simulink model "threelevel_evenorderel_SVPWM_working"  (R2016a)
settings: Solver=VariableStepAuto  StartTime=0.0  StopTime=0.1  RelTol=1e-3
libraries: powerlib x33, simulink x7
(part 2 of 2)

== matlab function threelevel_evenorderel_SVPWM_working/Ta, Tb, Tc calc1 ==
  data: Sa1 output; Sa2 output; Sb1 output; Sb2 output; Vd input; ma input; fundf input; swf input; time input; Sc1 output; Sc2 output
function [Sa1, Sa2, Sb1, Sb2, Sc1, Sc2] = fcn(Vd,ma,fundf, swf, time)
% this program works for magnitude of Vref is greater then Vd/3 meaning ma
% must be greater than 1/sqrt(3). for smaller ma's computation is a bit
% more tricky therefore it is omitted for simplicity for now. 
%#ok<*NASGU>
Vref = ma*Vd/sqrt(3); %magnitude of Vref
theta = 2*pi*fundf*time; %angle of Vref
angle = mod(theta, 2*pi);
Ts = 1/swf;
Ta = 0;
Tb = 0;
Tc = 0;
output = 0;
Sector1 = 0; Sector2 = 0; Sector3 = 0; Sector4= 0; Sector5 = 0; Sector6 = 0;
rgn2a = 0 ;rgn2b = 0; rgn3 = 0; rgn4 = 0;
Sa1=0; Sa2=0; Sa1P=0; Sa2P=0; Sb1=0; Sb2=0; Sb1P=0; Sb2P=0; Sc1=0; Sc2=0; Sc1P=0; Sc2P=0;
anglefrom3to2= 0 ;
timee = mod(time, Ts);

%% Sector 1


if (mod(theta, 2*pi)<=pi/3)&&(mod(theta, 2*pi)>0)  % sector 1

    n = 1;
    thetaprime = angle - (n-1)*pi/3;
        for aci = 0:0.00001:pi/3   
            la = sqrt(3)*cos(aci)-sin(aci);
                if (la*ma > 0.99)&&(la*ma<=1)
                    anglefrom3to2 = aci; %leaving angle from region 3 to region 2
                    break
                end
        end

    %anglefrom3to2 = asin(1-1/(sqrt(3)*ma)); 
    anglefrom2to4 = pi/3 - anglefrom3to2; %leaving angle from region 2 to region 4
    if (mod(theta, 2*pi)<=anglefrom3to2) % then sector 1 region 3
        rgn2a = 0 ;rgn2b = 0; rgn3 = 1; rgn4 = 0;
        Ta = Ts*(2-2*ma*sin(pi/3+thetaprime));
        Tb = Ts*2*ma*sin(thetaprime);
        Tc = Ts*(2*ma*sin(pi/3-thetaprime)-1);  
        times = [Tc/4 Tb/2 Ta/2 Tc/2 Ta/2 Tb/2 Tc/4];
        times = cumsum(times);
        va1 = [1 1 1 0 1 1 1];
        va2 = [1 1 1 1 1 1 1];
        vb1 = [0 0 0 0 0 0 0];
        vb2 = [1 1 0 0 0 1 1];
        vc1 = [0 0 0 0 0 0 0];
        vc2 = [1 0 0 0 0 0 1];
        for j = 1:7
            
            if(timee<times(j))
                break
            end
        end
        Sa1=va1(j); Sa2=va2(j);
        Sb1=vb1(j); Sb2=vb2(j); 
        Sc1=vc1(j); Sc2=vc2(j); 
    else if (mod(theta,2*pi)>anglefrom3to2)&&(mod(theta,2*pi)<=anglefrom2to4) % then sector 1 region 2
            if angle<= pi/6 % then 2a
                rgn2a= 1; rgn2b = 0; rgn3 = 0; rgn4=0;
            else % then 2b
                rgn2a= 0; rgn2b = 1; rgn3 = 0; rgn4=0;
            end
            Ta = Ts*(1-2*ma*sin(thetaprime));
            Tb = Ts*(2*ma*sin(pi/3+thetaprime)-1);
            Tc = Ts*(1-2*ma*sin(pi/3-thetaprime));  
            times = [Tc/4 Tb/2 Ta/2 Tc/2 Ta/2 Tb/2 Tc/4];
            times = cumsum(times);
        if(rgn2a)
            va1 = [1 1 0 0 0 1 1];
            va2 = [1 1 1 1 1 1 1];
            vb1 = [0 0 0 0 0 0 0];
            vb2 = [1 1 1 0 1 1 1];
            vc1 = [0 0 0 0 0 0 0];
            vc2 = [1 0 0 0 0 0 1];
        for j = 1:7
            if(timee<times(j))
                break
            end
        end
        Sa1=va1(j); Sa2=va2(j);
        Sb1=vb1(j); Sb2=vb2(j); 
        Sc1=vc1(j); Sc2=vc2(j); 
        end
        if(rgn2b)
            va1 = [0 1 1 1 1 1 0];
            va2 = [1 1 1 1 1 1 1];
            vb1 = [0 0 0 1 0 0 0];
            vb2 = [1 1 1 1 1 1 1];
            vc1 = [0 0 0 0 0 0 0];
            vc2 = [0 0 1 1 1 0 0];
        for j = 1:7
            if(timee<times(j))
                break
            end
        end
        Sa1=va1(j); Sa2=va2(j);
        Sb1=vb1(j); Sb2=vb2(j); 
        Sc1=vc1(j); Sc2=vc2(j);     
        end
            
        else if (mod(theta,2*pi)>anglefrom2to4) % then sector 1 region 4
               rgn2a = 0 ;rgn2b = 0; rgn3 = 0; rgn4 = 1;
               Ta = Ts*(2*ma*sin(thetaprime)-1);
               Tb = Ts*(2*ma*sin(pi/3-thetaprime));
               Tc = Ts*(2-2*ma*sin(pi/3+thetaprime));  
               times = [Tc/4 Tb/2 Ta/2 Tc/2 Ta/2 Tb/2 Tc/4];
               times = cumsum(times);
        va1 = [0 1 1 1 1 1 0];
        va2 = [1 1 1 1 1 1 1];
        vb1 = [0 0 1 1 1 0 0];
        vb2 = [1 1 1 1 1 1 1];
        vc1 = [0 0 0 0 0 0 0];
        vc2 = [0 0 0 1 0 0 0];
        for j = 1:7
            if(timee<times(j))
                break
            end
        end
        Sa1=va1(j); Sa2=va2(j);
        Sb1=vb1(j); Sb2=vb2(j); 
        Sc1=vc1(j); Sc2=vc2(j);
            end
        end
    end
    Sector1 = 1; Sector2 = 0; Sector3 = 0; Sector4= 0; Sector5 = 0; Sector6 = 0;
end
%% Sector 2


if (mod(theta, 2*pi)<=2*pi/3)&&(mod(theta, 2*pi)>pi/3)  % sector 2
    
    n = 2;
    thetaprime = angle - (n-1)*pi/3;
        for aci = 0:0.00001:pi/3   
            la = sqrt(3)*cos(aci)-sin(aci);
                if (la*ma > 0.99)&&(la*ma<=1)
                    anglefrom3to2 = aci+pi/3; %leaving angle from region 3 to region 2
                    break
                end
        end
    %anglefrom3to2 = pi/3 + asin(1-1/(sqrt(3)*ma));
    anglefrom2to4 = pi/3 + pi/3 - anglefrom3to2;
    if (mod(theta, 2*pi)<=anglefrom3to2) % then sector 2 region 3
        rgn2a = 0 ;rgn2b = 0; rgn3 = 1; rgn4 = 0;
        Ta = Ts*(2-2*ma*sin(pi/3+thetaprime));
        Tb = Ts*2*ma*sin(thetaprime);
        Tc = Ts*(2*ma*sin(pi/3-thetaprime)-1);
        times = [Tc/4 Tb/2 Ta/2 Tc/2 Ta/2 Tb/2 Tc/4];
        times = cumsum(times);
        va1 = [0 0 1 1 1 0 0];
        va2 = [1 1 1 1 1 1 1];
        vb1 = [0 1 1 1 1 1 0];
        vb2 = [1 1 1 1 1 1 1];
        vc1 = [0 0 0 0 0 0 0];
        vc2 = [0 0 0 1 0 0 0];
        for j = 1:7
            if(timee<times(j))
                break
            end
        end
        Sa1=va1(j); Sa2=va2(j);
        Sb1=vb1(j); Sb2=vb2(j); 
        Sc1=vc1(j); Sc2=vc2(j);
    else if (mod(theta,2*pi)>anglefrom3to2)&&(mod(theta,2*pi)<=anglefrom2to4) % then sector 2 region 2
            if angle<=pi/2 %then 2a
                rgn2a= 1; rgn2b = 0; rgn3 = 0; rgn4=0;
            else % then 2b
                rgn2a= 0; rgn2b = 1; rgn3 = 0; rgn4=0;
            end
            Ta = Ts*(1-2*ma*sin(thetaprime));
            Tb = Ts*(2*ma*sin(pi/3+thetaprime)-1);
            Tc = Ts*(1-2*ma*sin(pi/3-thetaprime)); 
            times = [Tc/4 Tb/2 Ta/2 Tc/2 Ta/2 Tb/2 Tc/4];
            times = cumsum(times);
        if(rgn2a)
            va1 = [0 0 0 1 0 0 0];
            va2 = [1 1 1 1 1 1 1];
            vb1 = [0 1 1 1 1 1 0];
            vb2 = [1 1 1 1 1 1 1];
            vc1 = [0 0 0 0 0 0 0];
            vc2 = [0 0 1 1 1 0 0];
        for j = 1:7
            if(timee<times(j))
                break
            end
        end
        Sa1=va1(j); Sa2=va2(j);
        Sb1=vb1(j); Sb2=vb2(j); 
        Sc1=vc1(j); Sc2=vc2(j); 
        end
        if(rgn2b)
            va1 = [0 0 0 0 0 0 0];
            va2 = [1 1 1 0 1 1 1];
            vb1 = [1 1 0 0 0 1 1];
            vb2 = [1 1 1 1 1 1 1];
            vc1 = [0 0 0 0 0 0 0];
            vc2 = [1 0 0 0 0 0 1];
        for j = 1:7
            if(timee<times(j))
                break
            end
        end
        Sa1=va1(j); Sa2=va2(j);
        Sb1=vb1(j); Sb2=vb2(j); 
        Sc1=vc1(j); Sc2=vc2(j);     
        end
        else if (mod(theta,2*pi)>anglefrom2to4) % then sector 2 region 4
               rgn2a = 0 ;rgn2b = 0; rgn3 = 0; rgn4 = 1;
               Ta = Ts*(2*ma*sin(thetaprime)-1);
               Tb = Ts*(2*ma*sin(pi/3-thetaprime));
               Tc = Ts*(2-2*ma*sin(pi/3+thetaprime));
               times = [Tc/4 Tb/2 Ta/2 Tc/2 Ta/2 Tb/2 Tc/4];
               times = cumsum(times);
        va1 = [0 0 0 0 0 0 0];
        va2 = [1 1 0 0 0 1 1];
        vb1 = [1 1 1 0 1 1 1];
        vb2 = [1 1 1 1 1 1 1];
        vc1 = [0 0 0 0 0 0 0];
        vc2 = [1 0 0 0 0 0 1];
        for j = 1:7
            if(timee<times(j))
                break
            end
        end
        Sa1=va1(j); Sa2=va2(j);
        Sb1=vb1(j); Sb2=vb2(j); 
        Sc1=vc1(j); Sc2=vc2(j);
            end
        end
    end
    Sector1 = 0; Sector2 = 1; Sector3 = 0; Sector4= 0; Sector5 = 0; Sector6 = 0;
end
%% Sector 3

if (mod(theta, 2*pi)<=pi)&&(mod(theta, 2*pi)>2*pi/3)  % sector 3
    
    n = 3;
    thetaprime = angle - (n-1)*pi/3;
        for aci = 0:0.00001:pi/3   
            la = sqrt(3)*cos(aci)-sin(aci);
                if (la*ma > 0.99)&&(la*ma<=1)
                    anglefrom3to2 = aci+pi/3+pi/3; %leaving angle from region 3 to region 2
                    break
                end
        end    
    %anglefrom3to2 = 2*pi/3 + asin(1-1/(sqrt(3)*ma));
    anglefrom2to4 = 2*pi/3 + pi/3 - anglefrom3to2;
    if (mod(theta, 2*pi)<=anglefrom3to2) % then sector 3 region 3
        rgn2a = 0 ;rgn2b = 0; rgn3 = 1; rgn4 = 0;
        Ta = Ts*(2-2*ma*sin(pi/3+thetaprime));
        Tb = Ts*2*ma*sin(thetaprime);
        Tc = Ts*(2*ma*sin(pi/3-thetaprime)-1); 
        times = [Tc/4 Tb/2 Ta/2 Tc/2 Ta/2 Tb/2 Tc/4];
        times = cumsum(times);
        va1 = [0 0 0 0 0 0 0];
        va2 = [1 0 0 0 0 0 1];
        vb1 = [1 1 1 0 1 1 1];
        vb2 = [1 1 1 1 1 1 1];
        vc1 = [0 0 0 0 0 0 0];
        vc2 = [1 1 0 0 0 1 1];
        for j = 1:7
            if(timee<times(j))
                break
            end
        end
        Sa1=va1(j); Sa2=va2(j);
        Sb1=vb1(j); Sb2=vb2(j); 
        Sc1=vc1(j); Sc2=vc2(j);
    else if (mod(theta,2*pi)>anglefrom3to2)&&(mod(theta,2*pi)<=anglefrom2to4) % then sector 3 region 2
            if angle<=5*pi/6 %then 2a
                rgn2a= 1; rgn2b = 0; rgn3 = 0; rgn4=0;
            else % then 2b
                rgn2a= 0; rgn2b = 1; rgn3 = 0; rgn4=0;
            end
            Ta = Ts*(1-2*ma*sin(thetaprime));
            Tb = Ts*(2*ma*sin(pi/3+thetaprime)-1);
            Tc = Ts*(1-2*ma*sin(pi/3-thetaprime));
            times = [Tc/4 Tb/2 Ta/2 Tc/2 Ta/2 Tb/2 Tc/4];
            times = cumsum(times);
            if(rgn2a)
            va1 = [0 0 0 0 0 0 0];
            va2 = [1 0 0 0 0 0 1];
            vb1 = [1 1 0 0 0 1 1];
            vb2 = [1 1 1 1 1 1 1];
            vc1 = [0 0 0 0 0 0 0];
            vc2 = [1 1 1 0 1 1 1];
        for j = 1:7
            if(timee<times(j))
                break
            end
        end
        Sa1=va1(j); Sa2=va2(j);
        Sb1=vb1(j); Sb2=vb2(j); 
        Sc1=vc1(j); Sc2=vc2(j); 
        end
        if(rgn2b)
            va1 = [0 0 0 0 0 0 0];
            va2 = [0 0 1 1 1 0 0];
            vb1 = [0 1 1 1 1 1 0];
            vb2 = [1 1 1 1 1 1 1];
            vc1 = [0 0 0 1 0 0 0];
            vc2 = [1 1 1 1 1 1 1];
        for j = 1:7
            if(timee<times(j))
                break
            end
        end
        Sa1=va1(j); Sa2=va2(j);
        Sb1=vb1(j); Sb2=vb2(j); 
        Sc1=vc1(j); Sc2=vc2(j);     
        end
        else if (mod(theta,2*pi)>anglefrom2to4) % then sector 3 region 4
                rgn2a = 0 ;rgn2b = 0; rgn3 = 0; rgn4 = 1;
               Ta = Ts*(2*ma*sin(thetaprime)-1);
               Tb = Ts*(2*ma*sin(pi/3-thetaprime));
               Tc = Ts*(2-2*ma*sin(pi/3+thetaprime));
               times = [Tc/4 Tb/2 Ta/2 Tc/2 Ta/2 Tb/2 Tc/4];
               times = cumsum(times);
        va1 = [0 0 0 0 0 0 0];
        va2 = [0 0 0 1 0 0 0];
        vb1 = [0 1 1 1 1 1 0];
        vb2 = [1 1 1 1 1 1 1];
        vc1 = [0 0 1 1 1 0 0];
        vc2 = [1 1 1 1 1 1 1];
        for j = 1:7
            if(timee<times(j))
                break
            end
        end
        Sa1=va1(j); Sa2=va2(j);
        Sb1=vb1(j); Sb2=vb2(j); 
        Sc1=vc1(j); Sc2=vc2(j);
            end
        end
    end
    Sector1 = 0; Sector2 = 0; Sector3 = 1; Sector4= 0; Sector5 = 0; Sector6 = 0;
end

%% Sector 4


if (mod(theta, 2*pi)<=4*pi/3)&&(mod(theta, 2*pi)>pi)  % sector 4
    

    n = 4;
    thetaprime = angle - (n-1)*pi/3;
        for aci = 0:0.00001:pi/3   
            la = sqrt(3)*cos(aci)-sin(aci);
                if (la*ma > 0.99)&&(la*ma<=1)
                    anglefrom3to2 = aci+pi/3+pi/3+pi/3; %leaving angle from region 3 to region 2
                    break
                end
        end    
    %anglefrom3to2 = pi + asin(1-1/(sqrt(3)*ma));
    anglefrom2to4 = pi + pi/3 - anglefrom3to2;
    if (mod(theta, 2*pi)<=anglefrom3to2) % then sector 4 region 3
        rgn2a = 0 ;rgn2b = 0; rgn3 = 1; rgn4 = 0;
        Ta = Ts*(2-2*ma*sin(pi/3+thetaprime));
        Tb = Ts*2*ma*sin(thetaprime);
        Tc = Ts*(2*ma*sin(pi/3-thetaprime)-1);
        times = [Tc/4 Tb/2 Ta/2 Tc/2 Ta/2 Tb/2 Tc/4];
        times = cumsum(times);
        va1 = [0 0 0 0 0 0 0];
        va2 = [0 0 0 1 0 0 0];
        vb1 = [0 0 1 1 1 0 0];
        vb2 = [1 1 1 1 1 1 1];
        vc1 = [0 1 1 1 1 1 0];
        vc2 = [1 1 1 1 1 1 1];
        for j = 1:7
            if(timee<times(j))
                break
            end
        end
        Sa1=va1(j); Sa2=va2(j);
        Sb1=vb1(j); Sb2=vb2(j); 
        Sc1=vc1(j); Sc2=vc2(j);
    else if (mod(theta,2*pi)>anglefrom3to2)&&(mod(theta,2*pi)<=anglefrom2to4) % then sector 4 region 2
            if angle<=7*pi/6 %then 2a
                rgn2a= 1; rgn2b = 0; rgn3 = 0; rgn4=0;
            else % then 2b
                rgn2a= 0; rgn2b = 1; rgn3 = 0; rgn4=0;
            end
            Ta = Ts*(1-2*ma*sin(thetaprime));
            Tb = Ts*(2*ma*sin(pi/3+thetaprime)-1);
            Tc = Ts*(1-2*ma*sin(pi/3-thetaprime));
            times = [Tc/4 Tb/2 Ta/2 Tc/2 Ta/2 Tb/2 Tc/4];
            times = cumsum(times);
             if(rgn2a)
            va1 = [0 0 0 0 0 0 0];
            va2 = [0 0 1 1 1 0 0];
            vb1 = [0 0 0 1 0 0 0];
            vb2 = [1 1 1 1 1 1 1];
            vc1 = [0 1 1 1 1 1 0];
            vc2 = [1 1 1 1 1 1 1];
        for j = 1:7
            if(timee<times(j))
                break
            end
        end
        Sa1=va1(j); Sa2=va2(j);
        Sb1=vb1(j); Sb2=vb2(j); 
        Sc1=vc1(j); Sc2=vc2(j); 
        end
        if(rgn2b)
            va1 = [0 0 0 0 0 0 0];
            va2 = [1 0 0 0 0 0 1];
            vb1 = [0 0 0 0 0 0 0];
            vb2 = [1 1 1 0 1 1 1];
            vc1 = [1 1 0 0 0 1 1];
            vc2 = [1 1 1 1 1 1 1];
        for j = 1:7
            if(timee<times(j))
                break
            end
        end
        Sa1=va1(j); Sa2=va2(j);
        Sb1=vb1(j); Sb2=vb2(j); 
        Sc1=vc1(j); Sc2=vc2(j);     
        end
        else if (mod(theta,2*pi)>anglefrom2to4) % then sector 4 region 4
                rgn2a = 0 ;rgn2b = 0; rgn3 = 0; rgn4 = 1;
               Ta = Ts*(2*ma*sin(thetaprime)-1);
               Tb = Ts*(2*ma*sin(pi/3-thetaprime));
               Tc = Ts*(2-2*ma*sin(pi/3+thetaprime));
               times = [Tc/4 Tb/2 Ta/2 Tc/2 Ta/2 Tb/2 Tc/4];
               times = cumsum(times);
               va1 = [0 0 0 0 0 0 0];
        va2 = [1 0 0 0 0 0 1];
        vb1 = [0 0 0 0 0 0 0];
        vb2 = [1 1 0 0 0 1 1];
        vc1 = [1 1 1 0 1 1 1];
        vc2 = [1 1 1 1 1 1 1];
        for j = 1:7
            if(timee<times(j))
                break
            end
        end
        Sa1=va1(j); Sa2=va2(j);
        Sb1=vb1(j); Sb2=vb2(j); 
        Sc1=vc1(j); Sc2=vc2(j);
            end
        end
    end
    Sector1 = 0; Sector2 = 0; Sector3 = 0; Sector4= 1; Sector5 = 0; Sector6 = 0;
end
%% Sector 5 

if (mod(theta, 2*pi)<=5*pi/3)&&(mod(theta, 2*pi)>4*pi/3)  % sector 5
    
    n = 5;
    thetaprime = angle - (n-1)*pi/3;
    %anglefrom3to2 = 4*pi/3 + asin(1-1/(sqrt(3)*ma));
        for aci = 0:0.00001:pi/3   
            la = sqrt(3)*cos(aci)-sin(aci);
                if (la*ma > 0.99)&&(la*ma<=1)
                    anglefrom3to2 = aci+pi/3+pi/3+pi/3+pi/3; %leaving angle from region 3 to region 2
                    break
                end
        end    
    anglefrom2to4 = 4*pi/3 + pi/3 - anglefrom3to2;
    if (mod(theta, 2*pi)<=anglefrom3to2) % then sector 5 region 3
        rgn2a = 0 ;rgn2b = 0; rgn3 = 1; rgn4 = 0;
        Ta = Ts*(2-2*ma*sin(pi/3+thetaprime));
        Tb = Ts*2*ma*sin(thetaprime);
        Tc = Ts*(2*ma*sin(pi/3-thetaprime)-1);
        times = [Tc/4 Tb/2 Ta/2 Tc/2 Ta/2 Tb/2 Tc/4];
            times = cumsum(times);
            va1 = [0 0 0 0 0 0 0];
        va2 = [1 1 0 0 0 1 1];
        vb1 = [0 0 0 0 0 0 0];
        vb2 = [1 0 0 0 0 0 1];
        vc1 = [1 1 1 0 1 1 1];
        vc2 = [1 1 1 1 1 1 1];
        for j = 1:7
            if(timee<times(j))
                break
            end
        end
        Sa1=va1(j); Sa2=va2(j);
        Sb1=vb1(j); Sb2=vb2(j); 
        Sc1=vc1(j); Sc2=vc2(j);
    else if (mod(theta,2*pi)>anglefrom3to2)&&(mod(theta,2*pi)<=anglefrom2to4) % then sector 5 region 2
            if angle<=3*pi/2 %then 2a
                rgn2a= 1; rgn2b = 0; rgn3 = 0; rgn4=0;
            else % then 2b
                rgn2a= 0; rgn2b = 1; rgn3 = 0; rgn4=0;
            end
            Ta = Ts*(1-2*ma*sin(thetaprime));
            Tb = Ts*(2*ma*sin(pi/3+thetaprime)-1);
            Tc = Ts*(1-2*ma*sin(pi/3-thetaprime));
            times = [Tc/4 Tb/2 Ta/2 Tc/2 Ta/2 Tb/2 Tc/4];
            times = cumsum(times);
            if(rgn2a)
            va1 = [0 0 0 0 0 0 0];
            va2 = [1 1 1 0 1 1 1];
            vb1 = [0 0 0 0 0 0 0];
            vb2 = [1 0 0 0 0 0 1];
            vc1 = [1 1 0 0 0 1 1];
            vc2 = [1 1 1 1 1 1 1];
        for j = 1:7
            if(timee<times(j))
                break
            end
        end
        Sa1=va1(j); Sa2=va2(j);
        Sb1=vb1(j); Sb2=vb2(j); 
        Sc1=vc1(j); Sc2=vc2(j); 
        end
        if(rgn2b)
            va1 = [0 0 0 1 0 0 0];
            va2 = [1 1 1 1 1 1 1];
            vb1 = [0 0 0 0 0 0 0];
            vb2 = [0 0 1 1 1 0 0];
            vc1 = [0 1 1 1 1 1 0];
            vc2 = [1 1 1 1 1 1 1];
        for j = 1:7
            if(timee<times(j))
                break
            end
        end
        Sa1=va1(j); Sa2=va2(j);
        Sb1=vb1(j); Sb2=vb2(j); 
        Sc1=vc1(j); Sc2=vc2(j);     
        end
        else if (mod(theta,2*pi)>anglefrom2to4) % then sector 5 region 4
               rgn2a = 0 ;rgn2b = 0; rgn3 = 0; rgn4 = 1;
               Ta = Ts*(2*ma*sin(thetaprime)-1);
               Tb = Ts*(2*ma*sin(pi/3-thetaprime));
               Tc = Ts*(2-2*ma*sin(pi/3+thetaprime)); 
               times = [Tc/4 Tb/2 Ta/2 Tc/2 Ta/2 Tb/2 Tc/4];
               times = cumsum(times);
               va1 = [0 0 1 1 1 0 0];
        va2 = [1 1 1 1 1 1 1];
        vb1 = [0 0 0 0 0 0 0];
        vb2 = [0 0 0 1 0 0 0];
        vc1 = [0 1 1 1 1 1 0];
        vc2 = [1 1 1 1 1 1 1];
        for j = 1:7
            if(timee<times(j))
                break
            end
        end
        Sa1=va1(j); Sa2=va2(j);
        Sb1=vb1(j); Sb2=vb2(j); 
        Sc1=vc1(j); Sc2=vc2(j);
            end
        end
    end
    Sector1 = 0; Sector2 = 0; Sector3 = 0; Sector4= 0; Sector5 = 1; Sector6 = 0;
end

%% Sector 6 

if (mod(theta, 2*pi)<=2*pi)&&(mod(theta, 2*pi)>5*pi/3)  % sector 6
    
    n = 6;
    thetaprime = angle - (n-1)*pi/3;
        for aci = 0:0.00001:pi/3   
            la = sqrt(3)*cos(aci)-sin(aci);
                if (la*ma > 0.99)&&(la*ma<=1)
                    anglefrom3to2 = aci+pi/3+pi/3+pi/3+pi/3+pi/3; %leaving angle from region 3 to region 2
                    break
                end
        end    
    %anglefrom3to2 = 5*pi/3 + asin(1-1/(sqrt(3)*ma));
    anglefrom2to4 = 5*pi/3 + pi/3 - anglefrom3to2;
    if (mod(theta, 2*pi)<=anglefrom3to2) % then sector 6 region 3
        rgn2a = 0 ;rgn2b = 0; rgn3 = 1; rgn4 = 0;
        Ta = Ts*(2-2*ma*sin(pi/3+thetaprime));
        Tb = Ts*2*ma*sin(thetaprime);
        Tc = Ts*(2*ma*sin(pi/3-thetaprime)-1);
        times = [Tc/4 Tb/2 Ta/2 Tc/2 Ta/2 Tb/2 Tc/4];
        times = cumsum(times);
        va1 = [0 1 1 1 1 1 0];
        va2 = [1 1 1 1 1 1 1];
        vb1 = [0 0 0 0 0 0 0];
        vb2 = [0 0 0 1 0 0 0];
        vc1 = [0 0 1 1 1 0 0];
        vc2 = [1 1 1 1 1 1 1];
        for j = 1:7
            if(timee<times(j))
                break
            end
        end
        Sa1=va1(j); Sa2=va2(j);
        Sb1=vb1(j); Sb2=vb2(j); 
        Sc1=vc1(j); Sc2=vc2(j);
        
    else if (mod(theta,2*pi)>anglefrom3to2)&&(mod(theta,2*pi)<=anglefrom2to4) % then sector 6 region 2
            if angle<=11*pi/6 %then 2a
                rgn2a= 1; rgn2b = 0; rgn3 = 0; rgn4=0;
            else % then 2b
                rgn2a= 0; rgn2b = 1; rgn3 = 0; rgn4=0;
            end
            Ta = Ts*(1-2*ma*sin(thetaprime));
            Tb = Ts*(2*ma*sin(pi/3+thetaprime)-1);
            Tc = Ts*(1-2*ma*sin(pi/3-thetaprime));
            times = [Tc/4 Tb/2 Ta/2 Tc/2 Ta/2 Tb/2 Tc/4];
            times = cumsum(times);
            if(rgn2a)
            va1 = [0 1 1 1 1 1 0];
            va2 = [1 1 1 1 1 1 1];
            vb1 = [0 0 0 0 0 0 0];
            vb2 = [0 0 1 1 1 0 0];
            vc1 = [0 0 0 1 0 0 0];
            vc2 = [1 1 1 1 1 1 1];
        for j = 1:7
            if(timee<times(j))
                break
            end
        end
        Sa1=va1(j); Sa2=va2(j);
        Sb1=vb1(j); Sb2=vb2(j); 
        Sc1=vc1(j); Sc2=vc2(j); 
        end
        if(rgn2b)
            va1 = [1 1 0 0 0 1 1];
            va2 = [1 1 1 1 1 1 1];
            vb1 = [0 0 0 0 0 0 0];
            vb2 = [1 0 0 0 0 0 1];
            vc1 = [0 0 0 0 0 0 0];
            vc2 = [1 1 1 0 1 1 1];
        for j = 1:7
            if(timee<times(j))
                break
            end
        end
        Sa1=va1(j); Sa2=va2(j);
        Sb1=vb1(j); Sb2=vb2(j); 
        Sc1=vc1(j); Sc2=vc2(j);     
        end
        else if (mod(theta,2*pi)>anglefrom2to4) % then sector 6 region 4
               rgn2a = 0 ;rgn2b = 0; rgn3 = 0; rgn4 = 1;
               Ta = Ts*(2*ma*sin(thetaprime)-1);
               Tb = Ts*(2*ma*sin(pi/3-thetaprime));
               Tc = Ts*(2-2*ma*sin(pi/3+thetaprime));
               times = [Tc/4 Tb/2 Ta/2 Tc/2 Ta/2 Tb/2 Tc/4];
               times = cumsum(times);
               va1 = [1 1 1 0 1 1 1];
        va2 = [1 1 1 1 1 1 1];
        vb1 = [0 0 0 0 0 0 0];
        vb2 = [1 0 0 0 0 0 1];
        vc1 = [0 0 0 0 0 0 0];
        vc2 = [1 1 0 0 0 1 1];
        for j = 1:7
            if(timee<times(j))
                break
            end
        end
        Sa1=va1(j); Sa2=va2(j);
        Sb1=vb1(j); Sb2=vb2(j); 
        Sc1=vc1(j); Sc2=vc2(j);
            end
        end
    end
    Sector1 = 0; Sector2 = 0; Sector3 = 0; Sector4= 0; Sector5 = 0; Sector6 = 1;
end
